simulink model "aerosim_simulink_fmu_1DOF_dynamics"  (R2024a)
settings: Solver=FixedStepAuto  StartTime=0.0  StopTime=inf  FixedStep=0.001  RelTol=1e-3
PreLoadFcn:
  | pos_x_init = 0.0;
  | pos_y_init = 0.0;
  | pos_z_init = 0.0;
  | Cd = 0.3;
  | A = 1.0;
  | z_ground = 0.0;
libraries: shared6dof x1
settings Model: Creator=ed  LastModifiedBy=Leo.Wong

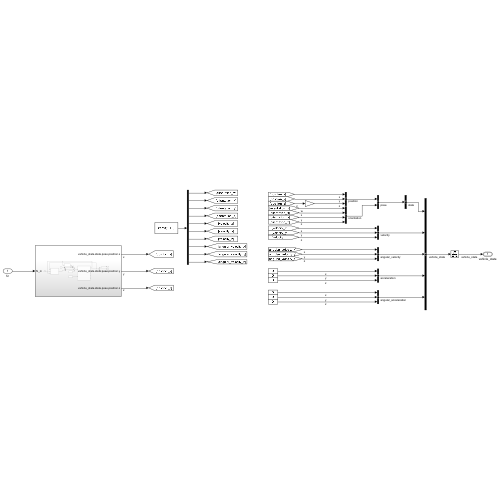
[thumbnail: Simulink's stored preview of the top-level diagram]
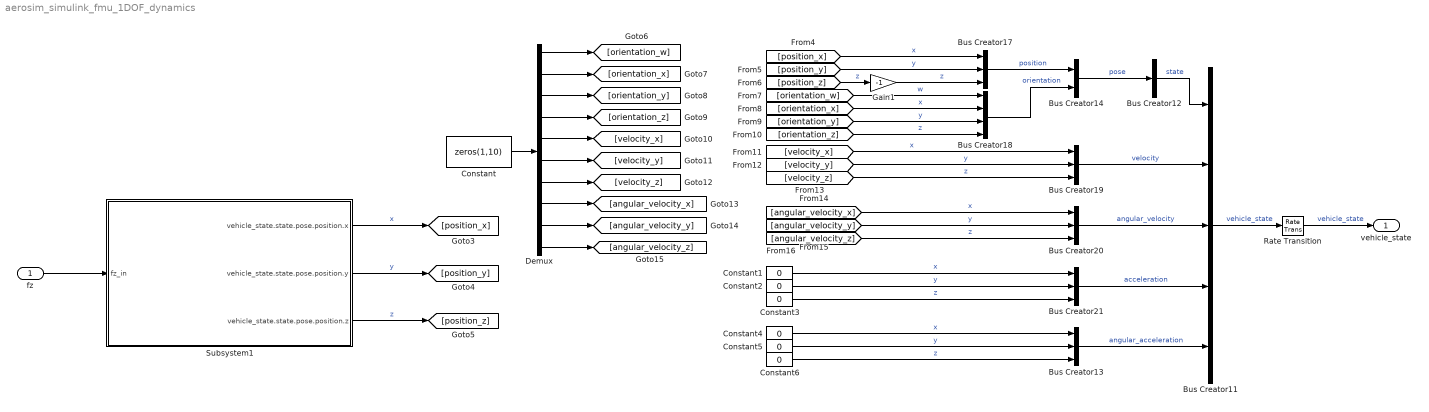
== system aerosim_simulink_fmu_1DOF_dynamics ==
  fz : Inport
  Bus Creator11 : BusCreator  Inputs=5  OutDataTypeStr=Bus: vehicle_state
  Bus Creator12 : BusCreator  Inputs=1  OutDataTypeStr=Bus: state
  Bus Creator13 : BusCreator  Inputs=3  OutDataTypeStr=Bus: angular_acceleration
  Bus Creator14 : BusCreator  Inputs=2  OutDataTypeStr=Bus: pose
  Bus Creator17 : BusCreator  Inputs=3  OutDataTypeStr=Bus: position
  Bus Creator18 : BusCreator  Inputs=4  OutDataTypeStr=Bus: orientation
  Bus Creator19 : BusCreator  Inputs=3  OutDataTypeStr=Bus: velocity
  Bus Creator20 : BusCreator  Inputs=3  OutDataTypeStr=Bus: angular_velocity
  Bus Creator21 : BusCreator  Inputs=3  OutDataTypeStr=Bus: acceleration
  Constant : Constant  Value=zeros(1,10)
  Constant{1..6} (6 alike) : Constant  Value=0  OutDataTypeStr=double
  Demux : Demux  Outputs=10
  Gain1 : Gain  Gain=-1
  Rate Transition : RateTransition  OutPortSampleTime=0.001
  Subsystem1 : Subsystem
  vehicle_state : Outport  OutDataTypeStr=Bus: vehicle_state
  wires:
  fz/1 -> Subsystem1/1(fz_in)
  Subsystem1/3(vehicle_state.state.pose.position.z) -> [position_z]  "z"
  Bus Creator21/1 -> Bus Creator11/4  "acceleration"
  Constant4/1 -> Bus Creator13/1  "x"
  [orientation_y] -> Bus Creator18/3  "y"
  Bus Creator12/1 -> Bus Creator11/1  "state"
  Bus Creator11/1 -> Rate Transition/1  "vehicle_state"
  Bus Creator20/1 -> Bus Creator11/3  "angular_velocity"
  Constant6/1 -> Bus Creator13/3  "z"
  Constant3/1 -> Bus Creator21/3  "z"
  Constant1/1 -> Bus Creator21/1  "x"
  [orientation_z] -> Bus Creator18/4  "z"
  Bus Creator19/1 -> Bus Creator11/2  "velocity"
  [velocity_z] -> Bus Creator19/3  "z"
  [angular_velocity_y] -> Bus Creator20/2  "y"
  Bus Creator13/1 -> Bus Creator11/5  "angular_acceleration"
  [angular_velocity_x] -> Bus Creator20/1  "x"
  [velocity_y] -> Bus Creator19/2  "y"
  Constant5/1 -> Bus Creator13/2  "y"
  [velocity_x] -> Bus Creator19/1  "x"
  [orientation_x] -> Bus Creator18/2  "x"
  Bus Creator14/1 -> Bus Creator12/1  "pose"
  [position_x] -> Bus Creator17/1  "x"
  [position_y] -> Bus Creator17/2  "y"
  Constant2/1 -> Bus Creator21/2  "y"
  [angular_velocity_z] -> Bus Creator20/3  "z"
  Bus Creator17/1 -> Bus Creator14/1  "position"
  [orientation_w] -> Bus Creator18/1  "w"
  Constant/1 -> Demux/1
  Demux/4 -> [orientation_z]
  Demux/3 -> [orientation_y]
  Demux/2 -> [orientation_x]
  Subsystem1/1(vehicle_state.state.pose.position.x) -> [position_x]  "x"
  Subsystem1/2(vehicle_state.state.pose.position.y) -> [position_y]  "y"
  Demux/5 -> [velocity_x]
  Demux/6 -> [velocity_y]
  Demux/7 -> [velocity_z]
  Demux/8 -> [angular_velocity_x]
  Demux/9 -> [angular_velocity_y]
  Demux/10 -> [angular_velocity_z]
  [position_z] -> Gain1/1  "z"
  Demux/1 -> [orientation_w]
  Gain1/1 -> Bus Creator17/3  "z"
  Rate Transition/1 -> vehicle_state/1  "vehicle_state"
  Bus Creator18/1 -> Bus Creator14/2  "orientation"

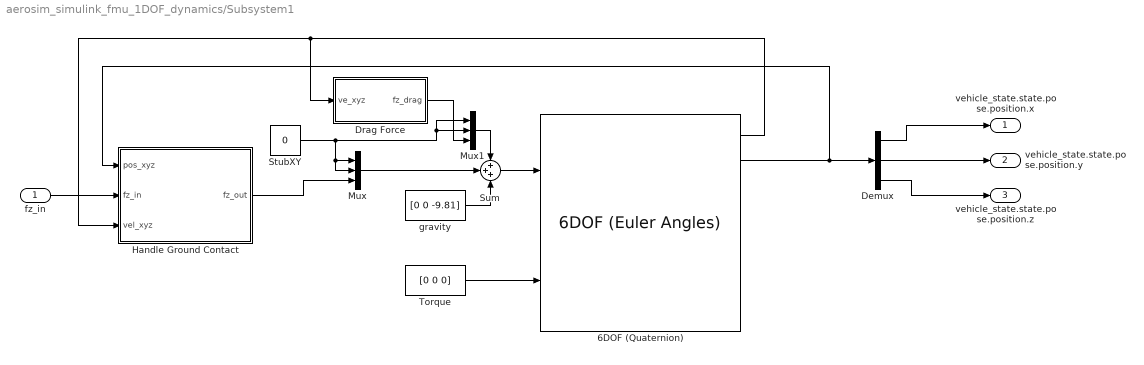
== system aerosim_simulink_fmu_1DOF_dynamics/Subsystem1 ==
  fz_in : Inport
  6DOF (Quaternion) : shared6dof/6DOF (Euler Angles)  units=Metric (MKS)  mtype=Fixed  rep=Quaternion  xme_0=[pos_x_init pos_y_init pos_z_init]  Vm_0=[0 0 0]  eul_0=[0 0 0]  pm_0=[0 0 0]  mass_0=1.0  mass_e=0.5  mass_f=2.0  inertia=eye(3)  inertia_e=eye(3)  inertia_f=2*eye(3)  k_quat=1.0  vre_flag=on  abi_flag=off  aMode=0  xme_statename=''  Vm_statename=''  eul_statename=''  quat_statename=''  pm_statename=''  mass_statename=''
      settings: LibrarySourceBlock=aerolib6dof2/6DOF (Quaternion)
  Demux : Demux  Outputs=3
  Drag Force : Subsystem
  Handle Ground Contact : Subsystem
  Mux : Mux  Inputs=3
  Mux1 : Mux  Inputs=3
  StubXY : Constant  Value=0
  Sum : Sum  Inputs=+++
  Torque : Constant  Value=[0 0 0]
  gravity : Constant  Value=[0 0 -9.81]
  vehicle_state.state.pose.position.x : Outport
  vehicle_state.state.pose.position.y : Outport  Port=2
  vehicle_state.state.pose.position.z : Outport  Port=3
  wires:
  Mux/1 -> Sum/2
  6DOF (Quaternion)/1 -> Handle Ground Contact/3(vel_xyz), Drag Force/1(ve_xyz)
  gravity/1 -> Sum/3
  Torque/1 -> 6DOF (Quaternion)/2
  6DOF (Quaternion)/2 -> Handle Ground Contact/1(pos_xyz), Demux/1
  StubXY/1 -> Mux1/2, Mux1/1, Mux/2, Mux/1
  Sum/1 -> 6DOF (Quaternion)/1
  Handle Ground Contact/1(fz_out) -> Mux/3
  fz_in/1 -> Handle Ground Contact/2(fz_in)
  Mux1/1 -> Sum/1
  Drag Force/1(fz_drag) -> Mux1/3
  Demux/3 -> vehicle_state.state.pose.position.z/1
  Demux/2 -> vehicle_state.state.pose.position.y/1
  Demux/1 -> vehicle_state.state.pose.position.x/1

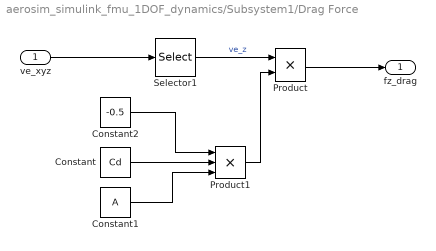
== system aerosim_simulink_fmu_1DOF_dynamics/Subsystem1/Drag Force ==
  ve_xyz : Inport
  Constant : Constant  Value=Cd
  Constant1 : Constant  Value=A
  Constant2 : Constant  Value=-0.5
  Product : Product
  Product1 : Product  Inputs=3
  Selector1 : Selector  InputPortWidth=3  IndexOptions=Index vector (dialog)  Indices=[3]  OutputSizes=1
  fz_drag : Outport
  wires:
  ve_xyz/1 -> Selector1/1
  Constant2/1 -> Product1/1
  Constant1/1 -> Product1/3
  Product1/1 -> Product/2
  Constant/1 -> Product1/2
  Product/1 -> fz_drag/1
  Selector1/1 -> Product/1  "ve_z"

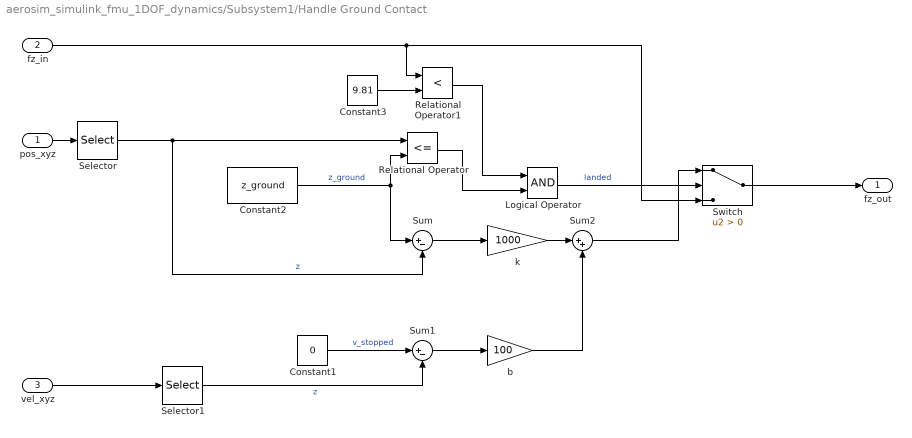
== system aerosim_simulink_fmu_1DOF_dynamics/Subsystem1/Handle Ground Contact ==
  pos_xyz : Inport
  fz_in : Inport  Port=2
  vel_xyz : Inport  Port=3
  Constant1 : Constant  Value=0
  Constant2 : Constant  Value=z_ground
  Constant3 : Constant  Value=9.81
  Logical Operator : Logic  AllPortsSameDT=off  OutDataTypeStr=boolean
  Relational Operator : RelationalOperator  Operator=<=  OutDataTypeStr=boolean  RndMeth=Simplest  InputSameDT=off
  Relational Operator1 : RelationalOperator  Operator=<  OutDataTypeStr=boolean  RndMeth=Simplest  InputSameDT=off
  Selector : Selector  InputPortWidth=3  IndexOptions=Index vector (dialog)  Indices=[3]  OutputSizes=1
  Selector1 : Selector  InputPortWidth=3  IndexOptions=Index vector (dialog)  Indices=[3]  OutputSizes=1
  Sum : Sum  Inputs=|+-
  Sum1 : Sum  Inputs=|+-
  Sum2 : Sum  Inputs=|++
  Switch : Switch  Criteria=u2 > Threshold  SaturateOnIntegerOverflow=off  InputSameDT=off
  b : Gain  Gain=100
  k : Gain  Gain=1000
  fz_out : Outport
  wires:
  Selector/1 -> Sum/2, Relational Operator/1  "z"
  Constant3/1 -> Relational Operator1/2
  Logical Operator/1 -> Switch/2  "landed"
  Relational Operator1/1 -> Logical Operator/1
  Constant2/1 -> Relational Operator/2, Sum/1  "z_ground"
  Relational Operator/1 -> Logical Operator/2
  fz_in/1 -> Switch/3, Relational Operator1/1
  Switch/1 -> fz_out/1
  pos_xyz/1 -> Selector/1
  Sum/1 -> k/1
  k/1 -> Sum2/1
  vel_xyz/1 -> Selector1/1
  Constant1/1 -> Sum1/1  "v_stopped"
  Selector1/1 -> Sum1/2  "z"
  Sum1/1 -> b/1
  b/1 -> Sum2/2
  Sum2/1 -> Switch/1
